simulink model "untitled3"  (R2023b)
settings: Solver=VariableStepAuto  StartTime=0.0  StopTime=10.0  RelTol=1e-3
settings Model: Creator=samee  LastModifiedBy=samee

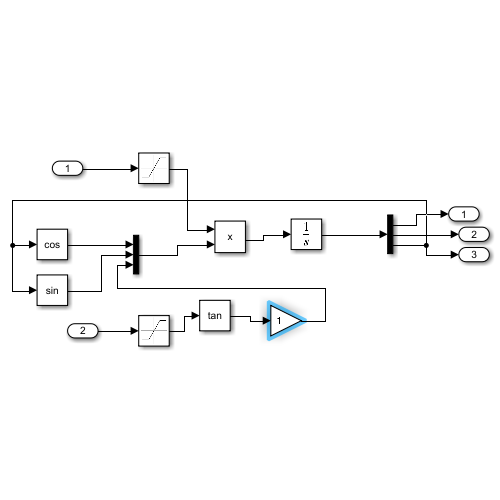
[thumbnail: Simulink's stored preview of the top-level diagram]
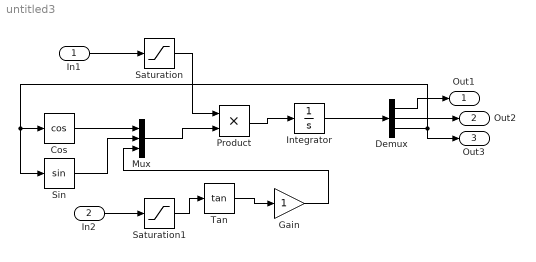
== system untitled3 ==
  In1 : Inport
  In2 : Inport  Port=2
  Cos : Trigonometry  Operator=cos
  Demux : Demux  Outputs=3
  Gain : Gain
  Integrator : Integrator
  Mux : Mux  Inputs=3
  Product : Product
  Saturation : Saturate
  Saturation1 : Saturate
  Sin : Trigonometry
  Tan : Trigonometry  Operator=tan
  Out1 : Outport
  Out2 : Outport  Port=2
  Out3 : Outport  Port=3
  wires:
  In1/1 -> Saturation/1
  Saturation/1 -> Product/1
  Product/1 -> Integrator/1
  Integrator/1 -> Demux/1
  Mux/1 -> Product/2
  Demux/1 -> Out1/1
  Demux/3 -> Out3/1, Sin/1, Cos/1
  Demux/2 -> Out2/1
  Cos/1 -> Mux/1
  Sin/1 -> Mux/2
  In2/1 -> Saturation1/1
  Saturation1/1 -> Tan/1
  Tan/1 -> Gain/1
  Gain/1 -> Mux/3
